simulink model "Motor_Simulation"  (R2025b)
settings: Solver=FixedStepAuto  StartTime=0.0  StopTime=inf  FixedStep=0.0001  RelTol=1e-3  EnableMultiTasking=on
libraries: slpidlib x1, raspberrypiNetworklib x1
settings Model: SimulationMode=external  ExtModeTrigDuration=2  Creator=jujma  LastModifiedBy=jujma
settings SolverCC: PositivePriorityOrder=on  AutoInsertRateTranBlk=on
settings OptimizationCC: EnhancedBackFolding=on  PassReuseOutputArgsAs=Individual arguments  ZeroExternalMemoryAtStartup=off  ZeroInternalMemoryAtStartup=off  MaxStackSize=200000  OptimizeBlockOrder=speed  DifferentSizesBufferReuse=on  OptimizationCustomize=off  EfficientTunableParamExpr=on
settings DebuggingCC: ParameterTunabilityLossMsg=error
settings HardwareCC: ProdBitPerPointer=32.0  ProdBitPerSizeT=32.0  ProdBitPerPtrDiffT=32.0  ProdLargestAtomicInteger=Long  ProdLargestAtomicFloat=Double  ProdWordSize=32.0  ProdLongLongMode=on  ProdHWDeviceType=ARM Compatible->ARM Cortex-A (32-bit)
settings RTWCC: SystemTargetFile=ert.tlc  HardwareBoard=Raspberry Pi  TLCOptions="-aInlineSetEventsForThisBaseRateFcn=TLC_FALSE -aSuppressMultiTaskScheduler=TLC_FALSE  -aRateBasedStepFcn=0"  TemplateMakefile=ert_default_tmf  Toolchain=GNU GCC Embedded Linux  BuildConfiguration=Faster Runs  Description=Embedded Coder
settings CodeAppCC: ForceParamTrailComments=on  IgnoreCustomStorageClasses=off  OperatorAnnotations=on  SimulinkDataObjDesc=on  SFDataObjDesc=on  InsertBlockDesc=on
settings ERTTargetCC: ExtModeTransport=2.0  ExtModeStaticAlloc=on  ExtModeMexFile=ext_xcp  ExtModeIntrfLevel=Level2 - Open  InlinedParameterPlacement=Hierarchical  CodeReplacementLibrary=ARM Cortex-A CMSIS  SupportContinuousTime=on  SupportVariableSizeSignals=on

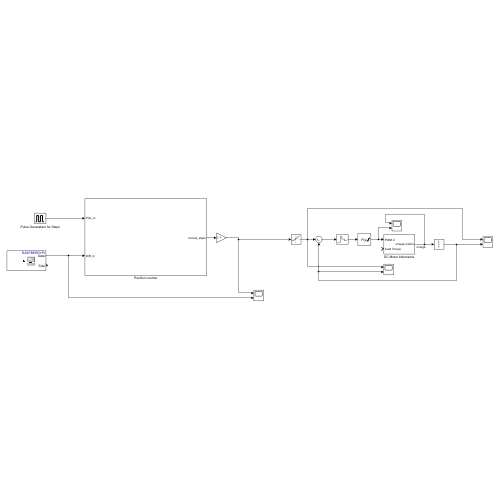
[thumbnail: Simulink's stored preview of the top-level diagram]
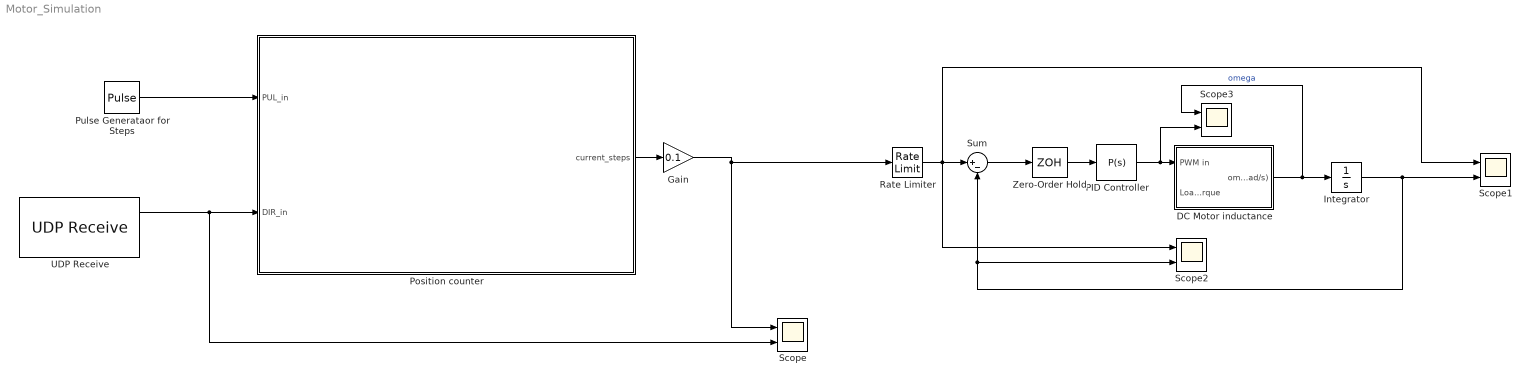
== system Motor_Simulation ==
  DC Motor inductance : Subsystem
  Gain : Gain  Gain=0.1
  Integrator : Integrator
  PID Controller : slpidlib/PID Controller  Controller=P  Form=Parallel  TimeDomain=Continuous-time  UseExternalTs=off  SampleTime=-1  IntegratorMethod=Forward Euler  FilterMethod=Forward Euler  ControllerParametersSource=internal  P=0.01  I=1  UseKiTs=off  D=0  UseExternalDerivativeSource=off  N=100  UseFilter=on  TunerSelectOption=Transfer Function Based (PID Tuner App)  InitialConditionSource=internal  InitialConditionForIntegrator=0  InitialConditionForFilter=0  DifferentiatorICPrevScaledInput=0  ExternalReset=none  TrackingMode=off  Kt=1  LimitOutput=on  SatLimitsSource=internal  UpperSaturationLimit=1  LowerSaturationLimit=-1  LinearizeAsGain=on  AntiWindupMode=none  Kb=1  LimitIntegrator=off  UpperIntegratorSaturationLimit=inf  LowerIntegratorSaturationLimit=-inf  POutMin=[]  POutMax=[]  IOutMin=[]  IOutMax=[]  DOutMin=[]  DOutMax=[]  NOutMin=[]  NOutMax=[]  SumOutMin=[]  SumOutMax=[]  SaturationOutMin=[]  SaturationOutMax=[]  PParamMin=[]  PParamMax=[]  IParamMin=[]  IParamMax=[]  DParamMin=[]  DParamMax=[]  NParamMin=[]  NParamMax=[]  KbParamMin=[]  KbParamMax=[]  KtParamMin=[]  KtParamMax=[]  KbOutMin=[]  KbOutMax=[]  KtOutMin=[]  KtOutMax=[]  IntegratorOutMin=[]  IntegratorOutMax=[]  FilterOutMin=[]  FilterOutMax=[]  SumI1OutMin=[]  SumI1OutMax=[]  SumI2OutMin=[]  SumI2OutMax=[]  SumI3OutMin=[]  SumI3OutMax=[]  SumI4OutMin=[]  SumI4OutMax=[]  SumDOutMin=[]  SumDOutMax=[]  DifferentiatorOutMin=[]  DifferentiatorOutMax=[]  FilterDiffOutCoefMin=[]  FilterDiffOutCoefMax=[]  ReciprocalOutMin=[]  ReciprocalOutMax=[]  SumDenOutMin=[]  SumDenOutMax=[]  SumNumOutMin=[]  SumNumOutMax=[]  DivideOutMin=[]  DivideOutMax=[]  UdiffTsProdOutMin=[]  UdiffTsProdOutMax=[]  NTsProdOutMin=[]  NTsProdOutMax=[]  UintegralTsProdOutMin=[]  UintegralTsProdOutMax=[]  UngainTsProdOutMin=[]  UngainTsProdOutMax=[]  ClampingZeroOutDataTypeStr=Inherit: Inherit via back propagation  ClampingZeroOutMin=[]  ClampingZeroOutMax=[]  FilterDenConstantOutDataTypeStr=Inherit: Inherit via back propagation  FilterDenConstantOutMin=[]  FilterDenConstantOutMax=[]  PCopyOutDataTypeStr=Inherit: Inherit via back propagation  PCopyOutMin=[]  PCopyOutMax=[]  NCopyOutDataTypeStr=Inherit: Inherit via back propagation  NCopyOutMin=[]  NCopyOutMax=[]  IntegratorContinuousStateAttributes=''  IntegratorStateMustResolveToSignalObject=off  IntegratorRTWStateStorageClass=Auto  FilterContinuousStateAttributes=''  FilterStateMustResolveToSignalObject=off  FilterRTWStateStorageClass=Auto  ParallelPVariant=InternalParameters  IdealPVariant=Disabled  IVariant=Disabled  DVariant=Disabled  IntegratorVariant=Disabled  SatVariant=Enabled  AWVariant=Disabled  PCopyVariant=Disabled  TRVariant=Disabled  FdbkBlocksVariant=Forward  IdealPFdbkVariant=Disabled  SatFdbkVariant=Disabled  DerivativeFilterVariant=Disabled  NVariant=Disabled  NCopyVariant=Disabled_SignalSpec  FilterICVariant=Disabled  IntegratorICVariant=Disabled  ExternalResetVariant=Disabled  TRSumVariant=Passthrough  SumFdbkVariant=Disabled  SumVariant=Passthrough_P  TsampFilterVariant=InternalTs  TsampNgainVariant=Passthrough  TsampIntegralVariant=Disabled_SignalSpec  ExternalSaturationOutDataTypeStr=Inherit: Same as second input  DerivativeSourceVariant=Disabled  PreIntVariant=InternalPreInt
  Position counter : Subsystem
  Pulse Generataor for Steps : DiscretePulseGenerator  PulseType=Time based  Period=0.01  PulseWidth=50
  Rate Limiter : RateLimiter  RisingSlewLimit=500  FallingSlewLimit=-500  SampleTimeMode=inherited
  Scope{,1..3} (4 alike) : Scope  NumInputPorts=2
      Scope settings: ActiveDisplayYMinimum=-32.587499999999991  ActiveDisplayYMaximum=283.2875
      Scope1 settings: ActiveDisplayYMinimum=-125.00000005212179  ActiveDisplayYMaximum=1125.0000004689507  DataLoggingVariableName=ScopeData4
      Scope2 settings: ActiveDisplayYMinimum=-124.99999999999997  ActiveDisplayYMaximum=1125  DataLoggingVariableName=ScopeData2
      Scope3 settings: ActiveDisplayYMinimum=283.88373980455344  ActiveDisplayYMaximum=538.39324107696757  DataLoggingVariableName=ScopeData5
  Sum : Sum  Inputs=|+-
  UDP Receive : raspberrypiNetworklib/UDP Receive  localURL='0.0.0.0'  localPort=55001  remoteURL='0.0.0.0'  remotePort=-1  recvBufferSize=8192  signalDatatype=double  dims=2  isVarSize=off  showBlockingTime=off  blockingTime=0  sampletime=0.0001  blockPlatform=Raspberry Pi
  Zero-Order Hold : ZeroOrderHold  SampleTime=0.1
  wires:
  Position counter/1(current_steps) -> Gain/1
  UDP Receive/1 -> Scope/2, Position counter/2(DIR_in)
  Pulse Generataor for Steps/1 -> Position counter/1(PUL_in)
  Integrator/1 -> Scope2/2, Sum/2, Scope1/2
  Sum/1 -> Zero-Order Hold/1
  Gain/1 -> Rate Limiter/1, Scope/1
  Zero-Order Hold/1 -> PID Controller/1
  Rate Limiter/1 -> Scope2/1, Scope1/1, Sum/1
  PID Controller/1 -> Scope3/2, DC Motor inductance/1(PWM in)
  DC Motor inductance/1(omega (rad/s)) -> Scope3/1, Integrator/1  "omega"

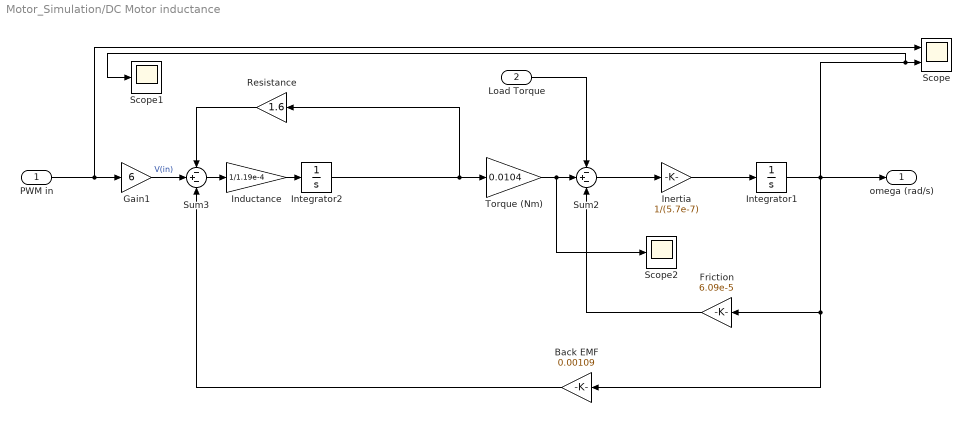
== system Motor_Simulation/DC Motor inductance ==
  PWM in : Inport
  Load Torque : Inport  Port=2
  Back EMF : Gain  Gain=0.00109
  Friction : Gain  Gain=6.09e-5
  Gain1 : Gain  Gain=6
  Inductance : Gain  Gain=1/1.19e-4
  Inertia : Gain  Gain=1/(5.7e-7)
  Integrator1 : Integrator
  Integrator2 : Integrator
  Resistance : Gain  Gain=1.6
  Scope : Scope  NumInputPorts=2
      settings: ActiveDisplayYMinimum=-0.12500005559101079  ActiveDisplayYMaximum=1.1250000061767791
  Scope1 : Scope
      settings: DataLoggingVariableName=ScopeData3
  Scope2 : Scope
      settings: ActiveDisplayYMinimum=-0.0048479602001581046  ActiveDisplayYMaximum=0.043631641801422948
  Sum2 : Sum  Inputs=-+-
  Sum3 : Sum  Inputs=-+-
  Torque (Nm) : Gain  Gain=0.0104
  omega (rad/s) : Outport
  wires:
  Back EMF/1 -> Sum3/3
  Resistance/1 -> Sum3/1
  Inertia/1 -> Integrator1/1
  Sum3/1 -> Inductance/1
  Friction/1 -> Sum2/3
  Sum2/1 -> Inertia/1
  Integrator1/1 -> Scope1/1, Scope/2, omega (rad/s)/1, Friction/1, Back EMF/1
  Inductance/1 -> Integrator2/1
  Torque (Nm)/1 -> Scope2/1, Sum2/2
  Load Torque/1 -> Sum2/1
  Gain1/1 -> Sum3/2  "V(in)"
  PWM in/1 -> Scope/1, Gain1/1
  Integrator2/1 -> Resistance/1, Torque (Nm)/1

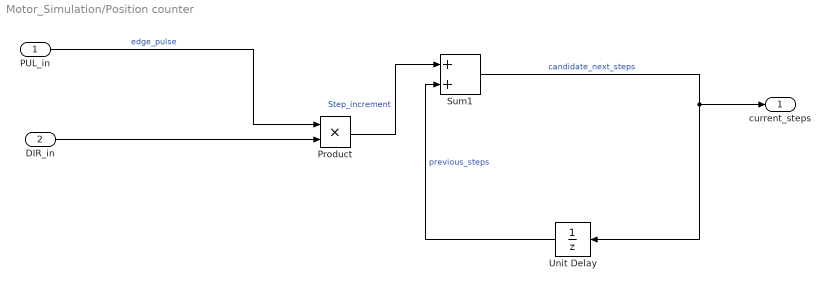
== system Motor_Simulation/Position counter ==
  PUL_in : Inport
  DIR_in : Inport  Port=2
  Product : Product
  Sum1 : Sum  Inputs=|++
  Unit Delay : UnitDelay  SampleTime=0.0001  HasFrameUpgradeWarning=on
  current_steps : Outport
  wires:
  PUL_in/1 -> Product/1  "edge_pulse"
  DIR_in/1 -> Product/2
  Product/1 -> Sum1/1  "Step_increment"
  Unit Delay/1 -> Sum1/2  "previous_steps"
  Sum1/1 -> Unit Delay/1, current_steps/1  "candidate_next_steps"
